simulink model "dyngeo"  (R2025b)
settings: Solver=VariableStepAuto  StartTime=0.0  StopTime=10.0  RelTol=1e-3
values from neighbouring files (symbols this model uses):
  g = 9.8    [initparams.m]
  I = diag([I_phi, I_theta, I_psi])    [initparams.m]
  m = 2.0    (= 2)    [initparams.m]
undefined symbols (not defined in the file or in its folder): Sim3dSensor
libraries: sim3dlib x2, uavsim3dlib x1, sim3dcameralib x1
settings Model: Creator=Sunetra  LastModifiedBy=Sunetra

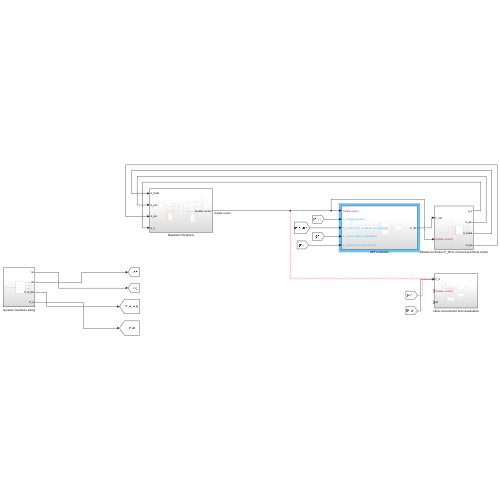
[thumbnail: Simulink's stored preview of the top-level diagram]
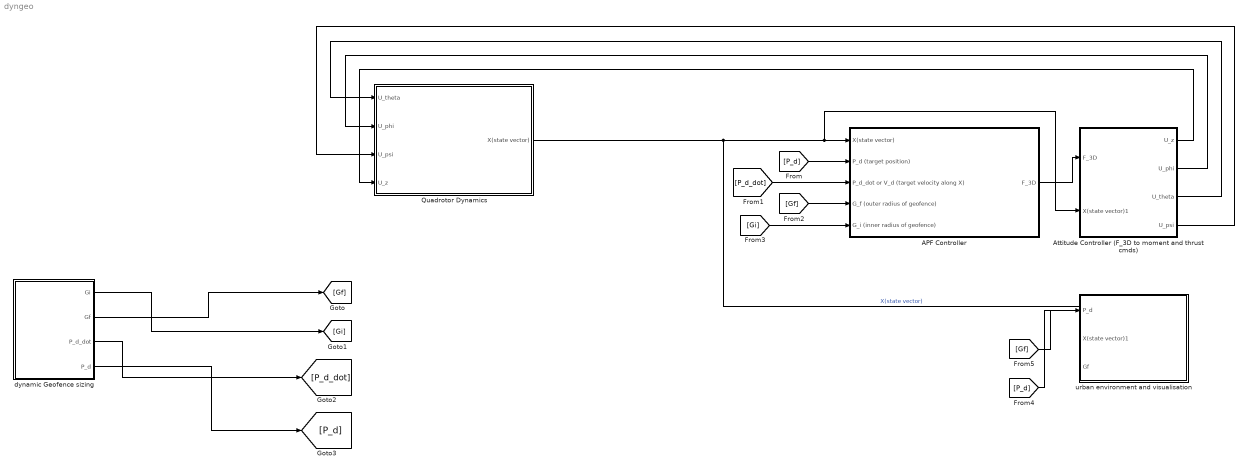
== system dyngeo ==
  APF Controller : Subsystem
  Attitude Controller (F_3D to moment and thrust cmds) : Subsystem
  Quadrotor Dynamics : Subsystem
  dynamic Geofence sizing : Subsystem
  urban environment and visualisation : Subsystem
  wires:
  Quadrotor Dynamics/1(X(state vector)) -> Attitude Controller (F_3D to moment and thrust cmds)/2(X(state vector)1), APF Controller/1(X(state vector))  "X(state vector)"
  APF Controller/1(F_3D) -> Attitude Controller (F_3D to moment and thrust cmds)/1(F_3D)
  Attitude Controller (F_3D to moment and thrust cmds)/1(U_z) -> Quadrotor Dynamics/4(U_z)
  Attitude Controller (F_3D to moment and thrust cmds)/2(U_phi) -> Quadrotor Dynamics/2(U_phi)
  Attitude Controller (F_3D to moment and thrust cmds)/3(U_theta) -> Quadrotor Dynamics/1(U_theta)
  Attitude Controller (F_3D to moment and thrust cmds)/4(U_psi) -> Quadrotor Dynamics/3(U_psi)
  dynamic Geofence sizing/2(Gf) -> [Gf]
  dynamic Geofence sizing/1(Gi) -> [Gi]
  dynamic Geofence sizing/3(P_d_dot) -> [P_d_dot]
  dynamic Geofence sizing/4(P_d) -> [P_d]
  [Gi] -> APF Controller/5(G_i (inner radius of geofence))
  [Gf] -> APF Controller/4(G_f (outer radius of geofence))
  [P_d_dot] -> APF Controller/3(P_d_dot or V_d (target velocity along X))
  [P_d] -> APF Controller/2(P_d (target position))
  [P_d] -> urban environment and visualisation/1(P_d)
  [Gf] -> ?

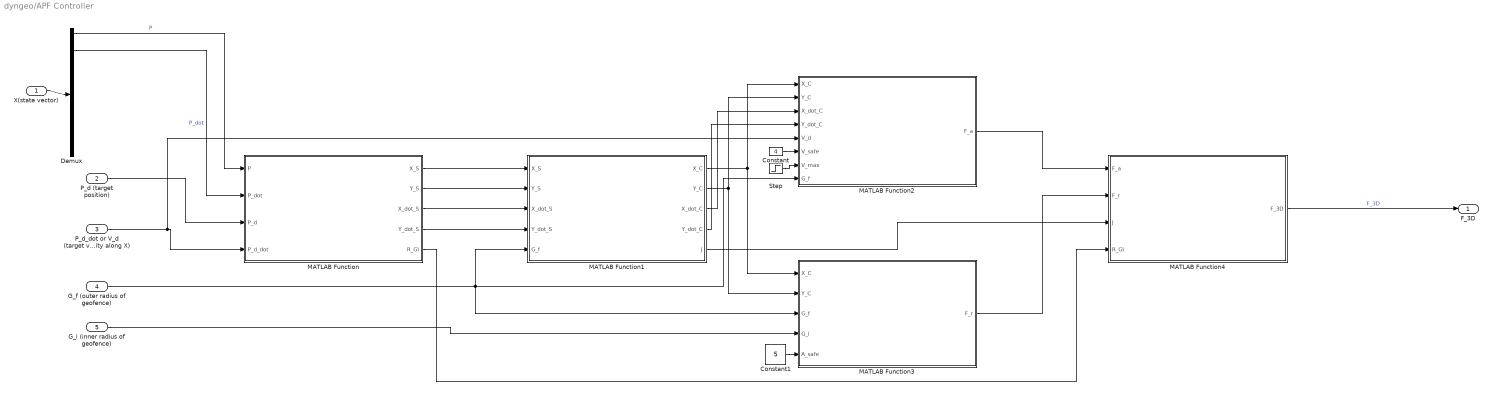
== system dyngeo/APF Controller ==
  X(state vector) : Inport
  P_d (target position) : Inport  Port=2
  P_d_dot or V_d (target velocity along X) : Inport  Port=3
  G_f (outer radius of geofence) : Inport  Port=4
  G_i (inner radius of geofence) : Inport  Port=5
  Constant : Constant  Value=4
  Constant1 : Constant  Value=5
  Demux : Demux  Outputs=[3, 3, 1, 1, 1, 1, 1, 1]
  MATLAB Function : MATLAB Function  TreatAsAtomicUnit=on
  MATLAB Function1 : MATLAB Function  TreatAsAtomicUnit=on
  MATLAB Function2 : MATLAB Function  TreatAsAtomicUnit=on
  MATLAB Function3 : MATLAB Function  TreatAsAtomicUnit=on
  MATLAB Function4 : MATLAB Function  TreatAsAtomicUnit=on
  Step : Step  Time=10  After=4  SampleTime=0
  F_3D : Outport
  wires:
  X(state vector)/1 -> Demux/1
  P_d (target position)/1 -> MATLAB Function/3(P_d)
  P_d_dot or V_d (target velocity along X)/1 -> MATLAB Function2/5(V_d), MATLAB Function/4(P_d_dot)
  Demux/1 -> MATLAB Function/1(P)  "P"
  Demux/2 -> MATLAB Function/2(P_dot)  "P_dot"
  MATLAB Function/1(X_S) -> MATLAB Function1/1(X_S)
  MATLAB Function/2(Y_S) -> MATLAB Function1/2(Y_S)
  MATLAB Function/3(X_dot_S) -> MATLAB Function1/3(X_dot_S)
  MATLAB Function/4(Y_dot_S) -> MATLAB Function1/4(Y_dot_S)
  G_f (outer radius of geofence)/1 -> MATLAB Function2/8(G_f), MATLAB Function3/3(G_f), MATLAB Function1/5(G_f)
  MATLAB Function1/1(X_C) -> MATLAB Function3/1(X_C), MATLAB Function2/1(X_C)
  MATLAB Function1/2(Y_C) -> MATLAB Function3/2(Y_C), MATLAB Function2/2(Y_C)
  MATLAB Function1/3(X_dot_C) -> MATLAB Function2/3(X_dot_C)
  MATLAB Function1/4(Y_dot_C) -> MATLAB Function2/4(Y_dot_C)
  G_i (inner radius of geofence)/1 -> MATLAB Function3/4(G_i)
  MATLAB Function2/1(F_a) -> MATLAB Function4/1(F_a)
  MATLAB Function3/1(F_r) -> MATLAB Function4/2(F_r)
  MATLAB Function1/5(J) -> MATLAB Function4/3(J)
  MATLAB Function/5(R_GI) -> MATLAB Function4/4(R_GI)
  MATLAB Function4/1(F_3D) -> F_3D/1  "F_3D"
  Constant/1 -> MATLAB Function2/6(V_safe)
  Step/1 -> MATLAB Function2/7(V_max)
  Constant1/1 -> MATLAB Function3/5(A_safe)

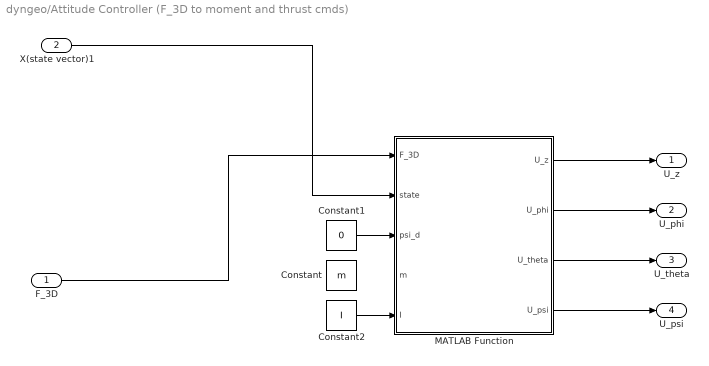
== system dyngeo/Attitude Controller (F_3D to moment and thrust cmds) ==
  F_3D : Inport
  X(state vector)1 : Inport  Port=2
  Constant : Constant  Value=m
  Constant1 : Constant  Value=0
  Constant2 : Constant  Value=I
  MATLAB Function : MATLAB Function  TreatAsAtomicUnit=on
  U_z : Outport
  U_phi : Outport  Port=2
  U_theta : Outport  Port=3
  U_psi : Outport  Port=4
  wires:
  F_3D/1 -> MATLAB Function/1(F_3D)
  X(state vector)1/1 -> MATLAB Function/2(state)
  Constant1/1 -> MATLAB Function/3(psi_d)
  Constant2/1 -> MATLAB Function/5(I)
  MATLAB Function/4(U_psi) -> U_psi/1
  MATLAB Function/3(U_theta) -> U_theta/1
  MATLAB Function/2(U_phi) -> U_phi/1
  MATLAB Function/1(U_z) -> U_z/1

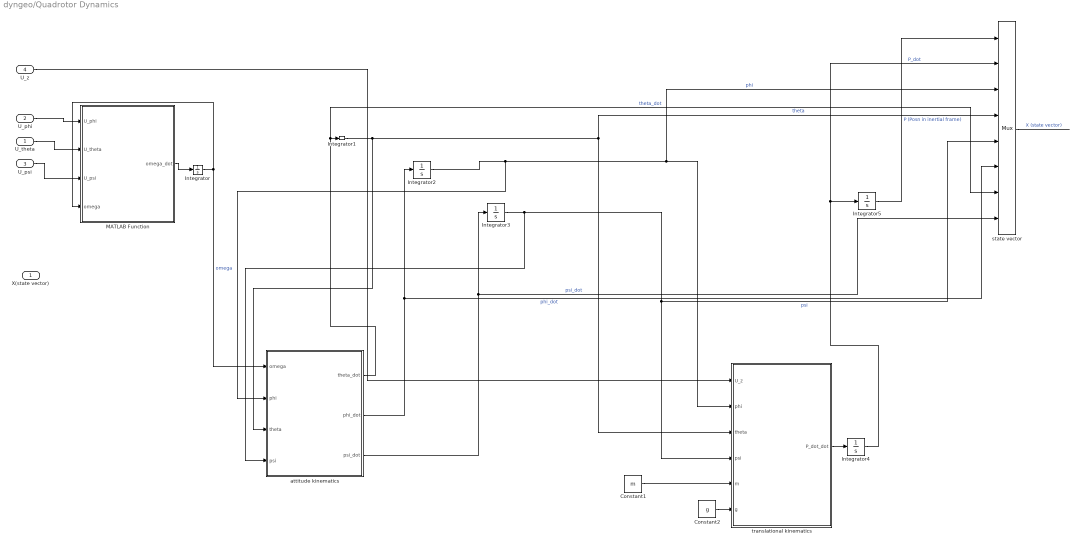
== system dyngeo/Quadrotor Dynamics ==
  U_theta : Inport
  U_phi : Inport  Port=2
  U_psi : Inport  Port=3
  U_z : Inport  Port=4
  Constant1 : Constant  Value=m
  Constant2 : Constant  Value=g
  Integrator : Integrator  InitialCondition=[0;0;0]
  Integrator{1..4} (4 alike) : Integrator
  Integrator5 : Integrator  InitialCondition=[0;0;0]
  MATLAB Function : MATLAB Function  TreatAsAtomicUnit=on
  attitude kinematics : MATLAB Function  TreatAsAtomicUnit=on
  "state vector " : Mux  Inputs=[3, 3, 1, 1, 1, 1, 1, 1]
  translational kinematics : MATLAB Function  TreatAsAtomicUnit=on
  X(state vector) : Outport
  wires:
  U_theta/1 -> MATLAB Function/2(U_theta)
  U_psi/1 -> MATLAB Function/3(U_psi)
  MATLAB Function/1(omega_dot) -> Integrator/1
  Integrator/1 -> MATLAB Function/4(omega), attitude kinematics/1(omega)  "omega"
  attitude kinematics/1(theta_dot) -> "state vector "/7, Integrator1/1  "theta_dot"
  attitude kinematics/2(phi_dot) -> Integrator2/1, "state vector "/6  "phi_dot"
  attitude kinematics/3(psi_dot) -> Integrator3/1, "state vector "/8  "psi_dot"
  Integrator2/1 -> attitude kinematics/2(phi), "state vector "/3, translational kinematics/2(phi)  "phi"
  Integrator3/1 -> attitude kinematics/4(psi), "state vector "/5, translational kinematics/4(psi)  "psi"
  Constant1/1 -> translational kinematics/5(m)
  Constant2/1 -> translational kinematics/6(g)
  translational kinematics/1(P_dot_dot) -> Integrator4/1
  Integrator4/1 -> "state vector "/2, Integrator5/1  "P_dot"
  Integrator5/1 -> "state vector "/1  "P (Posn in inertial frame)"
  Integrator1/1 -> attitude kinematics/3(theta), "state vector "/4, translational kinematics/3(theta)  "theta"
  U_phi/1 -> MATLAB Function/1(U_phi)
  U_z/1 -> translational kinematics/1(U_z)
  "state vector "/1 -> ?  "X (state vector)"

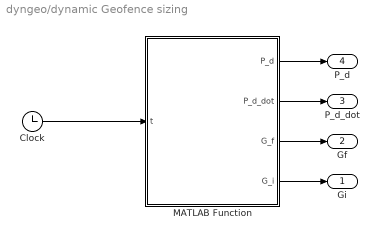
== system dyngeo/dynamic Geofence sizing ==
  Clock : Clock
  MATLAB Function : MATLAB Function  TreatAsAtomicUnit=on
  Gi : Outport
  Gf : Outport  Port=2
  P_d_dot : Outport  Port=3
  P_d : Outport  Port=4
  wires:
  Clock/1 -> MATLAB Function/1(t)
  MATLAB Function/1(P_d) -> P_d/1
  MATLAB Function/2(P_d_dot) -> P_d_dot/1
  MATLAB Function/3(G_f) -> Gf/1
  MATLAB Function/4(G_i) -> Gi/1

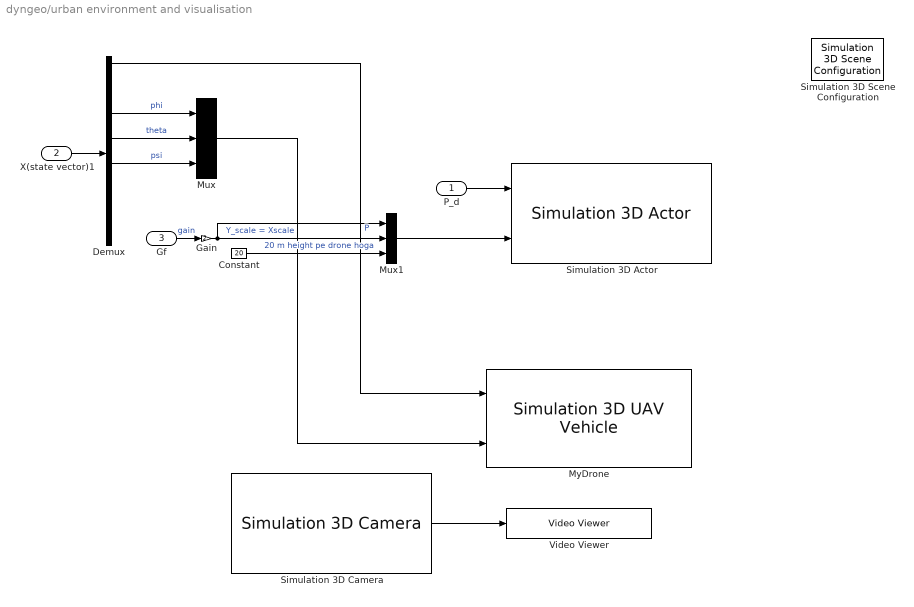
== system dyngeo/urban environment and visualisation ==
  P_d : Inport
  X(state vector)1 : Inport  Port=2
  Gf : Inport  Port=3
  Constant : Constant  Value=20
  Demux : Demux  Outputs=[3, 3, 1, 1, 1, 1, 1, 1]
  Gain : Gain  Gain=2
  Mux : Mux  Inputs=3
  Mux1 : Mux  Inputs=3
  MyDrone : uavsim3dlib/Simulation 3D UAV Vehicle  Priority=-1  Mesh=Quadrotor  MeshPath=/MathWorksUAVContent/UAVs/HexaRotorUAV/HexaRotor.HexaRotor  Color=Black  ActorName=MyDrone  UseGlobalFrame=off  InitialTranslation=[0 0 0]  InitialRotation=[0 0 0]  InitialTranslationGlobal=[0 0 0]  InitialGeoOrigin=[0 0 0]  InitialRotationGlobal=[0 0 0]  SampleTime=-1  ActorType=SimulinkVehicle  ID=C  aMode=4  ActorTag=MyDrone
  Simulation 3D Actor : sim3dlib/Simulation 3D Actor  Priority=1  ActorName=Sim3dActor1  ParentName=Scene Origin  Operation=Create at setup  InitScriptText=|  SampleTime=-1  Translation=[0 0 0]  Rotation=[0 0 0]  Scale=[1 1 1]  InputsText=Sim3dActor1.Translation Sim3dActor1.Scale  aMode=5  ActorTag=Sim3dActor1  ActorType=Sim3dActor  ID=1
      | % Reserved keywords:
      | % - Actor : handle to this actor object
      | % - World : handle to the world object
      | 
      | % Examples:
      | 
      | % Create a primitive geometry (optional)
      | % createShape(Actor, 'box', [1 1 1]);
      | 
      | % Initialize values (optional)
      | % Actor.Physics = true;
      | % Actor.Color = [1 0 0];
  Simulation 3D Camera : sim3dcameralib/Simulation 3D Camera  Priority=1  sensorTag=Sim3dSensor�  sensorId=1  sensorName=Sim3dSensor�  vehTagList={'MyDrone';'Scene Origin';'Sim3dActor1'}  vehTag=MyDrone  CoordinateSystem=ISO8855  mountLoc=Origin  offsetFlag=on  tmountOffset=[0, 0, 0]  extTmount=off  rmountOffset=[0, 0, 0]  extRmount=off  FocalLength=[1109, 1109]  OpticalCenter=[640, 360]  ImageSize=[720, 1280]  RadialDistortion=[0, 0]  TangentialDistortion=[0, 0]  SensorSkew=0  VisualizeFieldOfView=off  FieldOfViewRange=61  DepthOutportEnabled=off  SemanticOutportEnabled=off  TransformOutportEnabled=off  SampleTime=-1  mountPoint=[0 0 0]  mountOrientation=[0 0 0]  aMode=6  ID=1
      settings: LibrarySourceBlock=robotsim3dlib/Simulation 3D Camera
  Simulation 3D Scene Configuration : sim3dlib/Simulation 3D Scene Configuration  Priority=0  ProjectFormat=Default Scenes  SceneDesc=US city block  ProjectName=D:\MATLAb\toolbox\shared\sim3d_projects\automotive_project_windows\UE\WindowsNoEditor\VehicleSimulation.exe  ScenePath=/Game/Maps/HwStrght  EnableOpenDRIVE=off  vehTagList={'Custom';'MyDrone';'Scene Origin';'Sim3dActor1'}  vehTag=MyDrone  AttachedCameraRelativeTranslation=[0 0 0]  FreeCameraDefaultInitialTranslation=[-6, 0, 2]  AttachedCameraRelativeRotation=[0 0 0]  FreeCameraDefaultInitialRotation=[0, -15, 0]  ViewpointName=Custom  FreeCameraInitialTranslation=[-6, 0, 2]  ViewpointTranslation=[0 0 0]  FreeCameraInitialRotation=[0, -15, 0]  ViewpointRotation=[0 0 0]  OpVisEn=off  Ts=.02  EnableWindow=on  EnableRemoteAccess=off  EnableWeather=off  SunAzimuth=90  SunAltitude=40.0  EnableGeospatialSun=off  Latitude=0  Longitude=0  Date=2023-01-01  Time=10:30:00  GeoTimeZone=-5.0  SunDaylightSaving=off  wind=1  clouds=10  EnableVolumetricClouds=off  CloudCoverage=0  CloudAltitude=6  fog=0  rain=0  RaindropsEffect=off  SnowDensity=0  EnableGeospatial=off  TilesetSource=Earth terrain  UseTrueOrigin=off  OriginHeight=200  OriginLatitude=40.744652  OriginLongitude=-73.988864  MapStyle=Aerial  AdditionalAssetIDs=[]  UseAdvancedSunSky=off  SolarTime=11  TimeZone=-5  Day=21  Month=9  Year=2022  UseDaylightSavingTime=on  DSTStartDay=10  DSTStartMonth=3  DSTEndDay=3  DSTEndMonth=11  DSTSwitchHour=2  sensorTag=MainCamera1  sensorId=1  sensorName=MainCamera1  mountLoc=Origin  offsetFlag=off  tmountOffset=[0, 0, 0]  rmountOffset=[0, 0, 0]  HorizontalResolution=1280  VerticalResolution=720  HorizontalFOV=60  mountPoint=[0 0 0]  mountOrientation=[0 0 0]  aMode=0  ID=1  GeoTrigger=Inactive  ViewNameList={'Custom'}  ViewTranslationList={'[-6 0 2]'}  ViewRotationList={'[0 -15 0]'}
      settings: LibrarySourceBlock=aerolibsim3d/Simulation 3D Scene Configuration
  Video Viewer : VideoViewer  FigPos=[2041 741 418 304]
  wires:
  Demux/1 -> MyDrone/1  "P"
  X(state vector)1/1 -> Demux/1
  Demux/4 -> Mux/2  "theta"
  Demux/5 -> Mux/3  "psi"
  Demux/3 -> Mux/1  "phi"
  Mux/1 -> MyDrone/2
  P_d/1 -> Simulation 3D Actor/1
  Mux1/1 -> Simulation 3D Actor/2
  Gain/1 -> Mux1/2, Mux1/1  "Y_scale = Xscale"
  Constant/1 -> Mux1/3  "20 m height pe drone hoga"
  Gf/1 -> Gain/1  "gain"
  Simulation 3D Camera/1 -> Video Viewer/1

== matlab function dyngeo/APF Controller/MATLAB Function4 ==
  data: F_a input; F_3D output; F_r input; J input; R_GI input
function F_3D = inverse_mapping_2D23D(F_a, F_r, J, R_GI)
    % Inputs:
    % F_a, F_r : 2D force vectors from the Attractive and Repulsive fields
    % J        : 2x2 Jacobian matrix (from the Forward Mapping block)
    % R_GI     : 3x3 Rotation matrix (from the 3D to 2D Transform block)
    
    % Outputs:
    % F_3D     : 3x1 Commanded acceleration vector [U_x; U_y; U_z] in the inertial frame

    % 1. Calculate the net planar field
    F_planar = F_a + F_r;
    
    % 2. Invert the 2x2 Jacobian
    % We use a determinant check to prevent singular matrix errors 
    % at the extreme mathematical boundaries of the diffeomorphic map.
    if abs(det(J)) > 1e-6
        J_inv = inv(J);
    else
        J_inv = pinv(J); % Moore-Penrose pseudo-inverse as a numerical safety net
    end
    
    % 3. Construct the 3D Inverse Jacobian mapping (Equation 6)
    % The Z-axis remains unchanged (1) because the diffeomorphic map only squishes the X-Y plane
    J_inv_3D = [J_inv(1,1), J_inv(1,2), 0;
                J_inv(2,1), J_inv(2,2), 0;
                0,          0,          1];
                
    % 4. Pad the 2D planar force to 3D
    % The force is purely lateral in the cross-section, so Z is 0
    F_padded = [F_planar(1); F_planar(2); 0];
    
    % 5. Map the force back to the square cross-section
    F_square = J_inv_3D * F_padded;
    
    % 6. Rotate the force back to the 3D Inertial Frame (Equation 6)
    % Since R_GI is an orthogonal rotation matrix, its pseudo-inverse (dagger) 
    % is simply its transpose (R_GI').
    F_3D = R_GI' * F_square;
    
end

== matlab function dyngeo/Attitude Controller (F_3D to moment and thrust cmds)/MATLAB Function ==
  data: F_3D input; U_z output; state input; psi_d input; m input; I input; U_phi output; U_theta output; U_psi output
function [U_z, U_phi, U_theta, U_psi] = attitude_controller(F_3D, state, psi_d, m, I)
    % Inputs:
    % F_3D   : 3x1 Commanded acceleration vector from APF [U_x; U_y; U_z_accel]
    % state  : 12x1 State vector from Quadrotor [P; P_dot; phi; theta; psi; phi_dot; theta_dot; psi_dot]
    % psi_d  : Desired heading angle (rad)
    % m      : Mass (kg)
    % I      : 3x3 Inertia matrix
    
    % Outputs:
    % U_z    : Total thrust force command (N)
    % U_phi  : Roll moment command (Nm)
    % U_theta: Pitch moment command (Nm)
    % U_psi  : Yaw moment command (Nm)

    g = 9.8;

    % --- 1. Extract Current States ---
    % Assuming your state vector is packed as [P(1:3); P_dot(1:3); Euler(1:3); Euler_rates(1:3)]
    phi       = state(7);
    theta     = state(8);
    psi       = state(9);
    phi_dot   = state(10);
    theta_dot = state(11);
    psi_dot   = state(12);

    % --- 2. Force Allocation & Desired Angles (Eq A1 & A2) ---
    U_x = F_3D(1);
    U_y = F_3D(2);
    
    % Total thrust must counteract gravity and provide the Z acceleration
    U_z_accel = F_3D(3) + g; 
    
    % Convert commanded acceleration to total thrust force
    % We use max(0, ...) to ensure the drone cannot command "negative" pulling thrust
    U_z = m * max(0, U_z_accel);

    % Calculate desired roll and pitch angles to achieve U_x and U_y accelerations
    phi_d   = (U_x * sin(psi_d) - U_y * cos(psi_d)) / g;
    theta_d = (U_x * cos(psi_d) + U_y * sin(psi_d)) / g;

    % --- 3. PD Controller Gains ---
    % Sourced directly from the paper's tuning parameters
    
    % Roll and Pitch dynamics: damping ratio = 0.85, natural frequency = 14 rad/s
    zeta_rp = 0.85;
    wn_rp   = 14;
    
    % Yaw dynamics: damping ratio = 0.95, natural frequency = 18 rad/s
    zeta_y  = 0.95;
    wn_y    = 18;

    % --- 4. Calculate Control Moments (Eq A3) ---
    % U = Kp*(angle_d - angle) - Kv*(angle_dot)
    % where Kp = I * wn^2 and Kv = I * 2 * zeta * wn
    
    I_phi   = I(1,1);
    I_theta = I(2,2);
    I_psi   = I(3,3);

    % Roll Moment
    Kp_phi = I_phi * wn_rp^2;
    Kv_phi = I_phi * 2 * zeta_rp * wn_rp;
    U_phi  = Kp_phi * (phi_d - phi) - Kv_phi * phi_dot;

    % Pitch Moment
    Kp_theta = I_theta * wn_rp^2;
    Kv_theta = I_theta * 2 * zeta_rp * wn_rp;
    U_theta  = Kp_theta * (theta_d - theta) - Kv_theta * theta_dot;

    % Yaw Moment
    Kp_psi = I_psi * wn_y^2;
    Kv_psi = I_psi * 2 * zeta_y * wn_y;
    U_psi  = Kp_psi * (psi_d - psi) - Kv_psi * psi_dot;

end

== matlab function dyngeo/dynamic Geofence sizing/MATLAB Function ==
  data: t input; P_d output; P_d_dot output; G_f output; G_i output
function [P_d, P_d_dot, G_f, G_i] = mission_planner(t)

%To keep the model clean, this block will simultaneously calculate 
% the geofence sizes and generate the moving target position 
% (P_d) for the drone to chase.

%For this specific setup, the guidance logic simplifies significantly 
% because the path is a straight line. Since the curvature is zero, 
% you don't need the dynamic "breathing" behavior of the safety envelopes 
% that you would see during complex turns. Instead, the inner boundary 
% stays fixed relative to the outer boundary.

%For this initial setup, we will use the parameters 
% from Case 4 in the paper: a worst-case, head-on wind disturbance 
% ($\alpha_{max} = 180^\circ$) on a straight-line path. 
% Because a straight-line path has zero curvature, 
% the paper states (Equation 85) that the inner radius $G_i$ should simply 
% sit at $0.99 G_f$ to act as a static safety bumper, 
% rather than constantly expanding and shrinking.

% Inputs:
    % t       : Current simulation time (seconds)
    
    % Outputs:
    % P_d     : 3x1 Desired position vector
    % P_d_dot : 3x1 Desired velocity vector
    % G_f     : Outer geofence radius (m)
    % G_i     : Inner geofence radius (m)

    % --- 1. Mission & Wind Parameters (Case 4) ---
    V_d = 2.0;          % Desired flight speed (m/s)
    V_safe = 4.0;       % Drone's safe speed limit (m/s)
    V_max = 4.0;        % Max speed induced by worst-case wind (m/s)
    alpha_max = pi;     % Wind direction (180 deg = head-on wind)

    % APF Tuning Gains (sourced from paper)
    K_p = 0.0905;
    K_v = 0.4254;
    K_m = 1.0;          % Lyapunov stability gain

    % --- 2. Calculate Wind Perturbation (Equation 22) ---
    delta_V = sqrt((V_max*cos(alpha_max) - V_d)^2 + (V_max*sin(alpha_max))^2);

    % --- 3. Calculate Dynamic Shift Parameters ---
    K_a = V_max / V_d;
    mu = K_v / (K_p * K_a);

    % --- 4. Theorem 2: Geofence Sizing (Equations 20 & 21) ---
    % This calculates the minimum safe G_radius based on the Lyapunov bounds
    term1 = (K_m * delta_V^2 / K_v) / (1 + K_m / mu);
    term2 = mu * (V_safe - V_d);

    if sqrt(term1) < term2
        G_f = sqrt(term1);
    else
        % Eq 21: Expanding the quadratic root
        G_f = 0.5 * (-K_m*(V_safe - V_d) + sqrt((K_m*(V_safe - V_d))^2 + 4*(K_m*delta_V^2/K_v)));
    end

    % --- 5. Inner Radius (Equation 85 Logic) ---
    % For a straight path (curvature c(t) = 0), G_i is fixed near the outer wall
    G_i = 0.99 * G_f;

    % --- 6. Path Generation (Straight Line along X-axis) ---
    P_d = [V_d * t; 0; 0];
    P_d_dot = [V_d; 0; 0];
    
end

== matlab function dyngeo/Quadrotor Dynamics/attitude kinematics ==
  data: omega input; phi input; theta input; psi input; theta_dot output; phi_dot output; psi_dot output
function [theta_dot, phi_dot,psi_dot] = attitude_kinematics(omega,phi,theta, psi)

% Inputs:
    % omega : Angular velocity [p; q; r] (rad/s) in body frame
    % phi   : Roll angle (rad)
    % theta : Pitch angle (rad)
    % psi   : Yaw angle (rad)
    
    % Outputs:
    % phi_dot   : Roll rate (rad/s)
    % theta_dot : Pitch rate (rad/s)
    % psi_dot   : Yaw rate (rad/s)

    % Define the transformation matrix from Equation A5
    W = [cos(theta), 0, -cos(phi)*sin(theta);
         0,          1,  sin(phi);
         sin(theta), 0,  cos(phi)*cos(theta)];
         
    % Calculate Euler rates: [phi_dot; theta_dot; psi_dot] = W^-1 * omega
    % Using the backslash operator (\) for efficient matrix inversion
    euler_rates = W \ omega;
    
    % Extract individual rates for the output ports
    phi_dot   = euler_rates(1);
    theta_dot = euler_rates(2);
    psi_dot   = euler_rates(3);
end

== matlab function dyngeo/Quadrotor Dynamics/MATLAB Function ==
  data: U_phi input; omega_dot output; U_theta input; U_psi input; omega input
function omega_dot = rotational_dynamics(U_phi, U_theta, U_psi, omega)

    % Pull I directly from workspace as a parameter
    I = diag([0.0196, 0.0196, 0.0264]); % hardcode or match your workspace values

    omega = omega(:);  % ensure 3x1

    M = [U_phi; U_theta; U_psi];

    omega_dot = I \ (M - cross(omega, I * omega));
end

== matlab function dyngeo/Quadrotor Dynamics/translational kinematics ==
  data: U_z input; P_dot_dot output; phi input; theta input; psi input; m input; g input
function P_dot_dot   = translational_physics(U_z,phi, theta, psi, m, g)

% Inputs:
    % U_z   : Total thrust command (N)
    % phi   : Roll angle (rad)
    % theta : Pitch angle (rad)
    % psi   : Yaw angle (rad)
    % m     : Mass (kg) sourced from workspace
    % g     : Gravity (m/s^2) sourced from workspace
    
    % Outputs:
    % P_dot_dot : Linear acceleration [x_ddot; y_ddot; z_ddot] in inertial frame

    % 1. Construct the Z-Y-X Rotation Matrix (R^BN) from Equation A6
    % Row 1
    R11 = cos(theta)*cos(psi);
    R12 = cos(psi)*sin(theta)*sin(phi) - sin(psi)*cos(phi);
    R13 = cos(psi)*sin(theta)*cos(phi) + sin(psi)*sin(phi);
    
    % Row 2
    R21 = sin(psi)*cos(theta);
    R22 = sin(psi)*sin(theta)*sin(phi) + cos(psi)*cos(phi);
    R23 = sin(psi)*sin(theta)*cos(phi) - cos(psi)*sin(phi);
    
    % Row 3
    R31 = -sin(theta);
    R32 = cos(theta)*sin(phi);
    R33 = cos(theta)*cos(phi);
    
    R_BN = [R11, R12, R13; 
            R21, R22, R23; 
            R31, R32, R33];
            
    % 2. Implement Position Dynamics from Equation A7
    gravity_vector = [0; 0; -g];
    
    % The thrust acts purely along the body Z-axis.
    % Dividing U_z by m converts force (Newtons) to acceleration (m/s^2)
    thrust_vector = [0; 0; U_z / m]; 
    
    % Calculate final linear acceleration
    P_dot_dot = gravity_vector + (R_BN * thrust_vector);
end

== matlab function dyngeo/APF Controller/MATLAB Function ==
  data: P input; X_S output; P_dot input; P_d input; P_d_dot input; Y_S output; X_dot_S output; Y_dot_S output; R_GI output
function [X_S, Y_S, X_dot_S, Y_dot_S, R_GI] = frame_transform_3D_to_2D(P, P_dot, P_d, P_d_dot)
    % Inputs:
    % P, P_dot       : Current UAS 3D position and velocity (3x1 vectors)
    % P_d, P_d_dot   : Desired 3D position and velocity on the path (3x1 vectors)
    
    % Outputs:
    % X_S, Y_S       : 2D Relative position in the square cross-section
    % X_dot_S, Y_dot_S : 2D Relative velocity in the square cross-section
    % R_GI           : 3x3 Rotation matrix (Save this to map forces back to 3D later)

    % Ensure inputs are column vectors for matrix operations
    P = P(:); P_dot = P_dot(:); P_d = P_d(:); P_d_dot = P_d_dot(:);
    
    % 1. Calculate relative 3D position and velocity
    del_P = P - P_d;
    del_P_dot = P_dot - P_d_dot;
    
    % 2. Path tangent vector (X_hat) [cite: 299]
    v_d_norm = norm(P_d_dot);
    if v_d_norm > 1e-6
        X_hat = P_d_dot / v_d_norm;
    else
        X_hat = [1; 0; 0]; % Fallback if desired velocity drops to exact 0
    end
    
    % 3. Intermediate frame vectors (Y_i_hat, Z_i_hat) [cite: 300, 301]
    Y_i_hat = [0; 1; 0];
    cross_X_Yi = cross(X_hat, Y_i_hat);
    if norm(cross_X_Yi) > 1e-6
        Z_i_hat = cross_X_Yi / norm(cross_X_Yi);
    else
        Z_i_hat = [0; 0; 1]; % Fallback if path is perfectly vertical
        Y_i_hat = cross(Z_i_hat, X_hat);
    end
    
    % 4. Geofence frame vectors (Z_g_hat, Y_g_hat) [cite: 301, 302]
    cross_X_delP = cross(X_hat, del_P);
    
    % Singularity handling: If drone is exactly on the centerline, cross product is 0
    if norm(cross_X_delP) > 1e-6
        Z_g_hat = cross_X_delP / norm(cross_X_delP);
        Y_g_hat = cross(Z_g_hat, X_hat) / norm(cross(Z_g_hat, X_hat));
    else
        % Align Geofence frame with Intermediate frame to avoid divide-by-zero
        Z_g_hat = Z_i_hat;
        Y_g_hat = Y_i_hat;
    end
    
    % 5. Construct the Rotation Matrix [R_GI] (Equation 4) [cite: 306]
    e1 = [1; 0; 0];
    M_i = [e1, Y_i_hat, Z_i_hat];
    M_g = [X_hat, Y_g_hat, Z_g_hat];
    
    % R_GI = M_i * M_g^T
    R_GI = M_i * M_g'; 
    
    % 6. Apply rotation to get states in the square cross-section [cite: 306]
    P_S_3D = R_GI * del_P;
    P_S_dot_3D = R_GI * del_P_dot;
    
    % 7. Extract the 2D planar components (We only care about the X and Y plane here)
    X_S = P_S_3D(1);
    Y_S = P_S_3D(2);
    X_dot_S = P_S_dot_3D(1);
    Y_dot_S = P_S_dot_3D(2);
end

== matlab function dyngeo/APF Controller/MATLAB Function1 ==
  data: X_C output; X_S input; Y_S input; X_dot_S input; Y_dot_S input; Y_C output; X_dot_C output; Y_dot_C output; J output; G_f input
function [X_C, Y_C, X_dot_C, Y_dot_C, J] = square2circle(X_S, Y_S, X_dot_S, Y_dot_S, G_f)
    % Inputs:
    % X_S, Y_S         : 2D position in the square cross-section
    % X_dot_S, Y_dot_S : 2D velocity in the square cross-section
    % G_f              : Outer geofence radius (G_radius)
    
    % Outputs:
    % X_C, Y_C         : 2D position in the circular manifold
    % X_dot_C, Y_dot_C : 2D velocity in the circular manifold
    % J                : 2x2 Jacobian matrix (passed forward for inverse mapping)

    % 1. Implement Equation 2 (Elliptical Grid Mapping)
    % We use max(0, ...) to prevent imaginary numbers if floating-point 
    % inaccuracies push the drone slightly past the absolute corner.
    term_Y = max(0, 1 - 0.5 * (Y_S / G_f)^2);
    term_X = max(0, 1 - 0.5 * (X_S / G_f)^2);
    
    X_C = X_S * sqrt(term_Y);
    Y_C = Y_S * sqrt(term_X);
    
    % 2. Calculate the Jacobian Matrix elements for velocity mapping
    % J11 = d(X_C)/d(X_S)
    J11 = sqrt(term_Y);
    
    % J12 = d(X_C)/d(Y_S)
    if term_Y > 1e-6
        J12 = - (X_S * Y_S) / (2 * G_f^2 * sqrt(term_Y));
    else
        J12 = 0; % Prevent divide-by-zero at extreme boundaries
    end
    
    % J21 = d(Y_C)/d(X_S)
    if term_X > 1e-6
        J21 = - (X_S * Y_S) / (2 * G_f^2 * sqrt(term_X));
    else
        J21 = 0;
    end
    
    % J22 = d(Y_C)/d(Y_S)
    J22 = sqrt(term_X);
    
    % Construct the 2x2 Jacobian
    J = [J11, J12; 
         J21, J22];
         
    % 3. Map the velocities into the circular manifold using the Jacobian
    V_C = J * [X_dot_S; Y_dot_S];
    
    X_dot_C = V_C(1);
    Y_dot_C = V_C(2);
end

== matlab function dyngeo/APF Controller/MATLAB Function2 ==
  data: X_C input; F_a output; Y_C input; X_dot_C input; Y_dot_C input; V_d input; V_safe input; V_max input; G_f input
function F_a = attractive_field(X_C, Y_C, X_dot_C, Y_dot_C, V_d, V_safe, V_max, G_f)
    % Outputs:
    % F_a : 2D Attractive force vector in the circular manifold
    
    % Internal Proportional and Derivative Gains 
    % (You can tune these later or expose them as block inputs)
    K_p = 0.0905; 
    K_v = 0.4254; 

    % Drone state relative to the desired position (which sits at [0;0] in this frame)
    Q = [X_C; Y_C];
    Q_dot = [X_dot_C; Y_dot_C];
    norm_Q = norm(Q);

    % If the drone is outside the outer geofence, F_a is mathematically 0 
    % (The repulsive field handles the extreme edge)
    if norm_Q > G_f
        F_a = [0; 0];
        return;
    end

    % 1. Calculate dynamic shift parameters
    K_a = V_max / V_d;
    mu = K_v / (K_p * K_a);

    % Path tangent vector in this rotated 2D frame is strictly along the X-axis
    X_hat = [1; 0];

    % 2. Calculate the zero-potential point (Q_d)
    % Initial assumption for shift X_E (Equation 15)
    X_E = mu * V_d;
    Q_d = X_E * X_hat;
    dist_Q_Qd = norm(Q - Q_d);

    % Check if the drone crossed the velocity boundary
    if dist_Q_Qd > mu * V_safe
        % Recalculate X_E dynamically to prevent exceeding safe speeds
        X_E = V_d * dist_Q_Qd / V_safe;
        Q_d = X_E * X_hat;
    end

    % 3. Calculate Reference Velocity (Equation 9)
    Q_d_dot = (K_p / K_v) * (Q_d - Q);
    norm_Q_d_dot = norm(Q_d_dot);

    if norm_Q_d_dot > 1e-6
        gamma = min(K_a, V_safe / norm_Q_d_dot);
    else
        gamma = K_a;
    end

    % 4. Compute Final Attractive Force (Equation 10)
    F_a = -K_v * (Q_dot - gamma * Q_d_dot);
end

== matlab function dyngeo/APF Controller/MATLAB Function3 ==
  data: X_C input; F_r output; Y_C input; G_f input; G_i input; A_safe input
function F_r = repulsive_field(X_C, Y_C, G_f, G_i, A_safe)
    % Outputs:
    % F_r : 2D Repulsive force vector in the circular manifold
    
    % Eta defines the fraction of A_safe reserved for the attractive field.
    % We assume 50% is reserved for path curvature here (eta = 0.5).
    eta = 0.5; 

    % Position vector
    Q = [X_C; Y_C];
    norm_Q = norm(Q);

    % Calculate signed distances (Equation 48 & 49)
    rho_i = G_i - norm_Q;
    rho = G_f - norm_Q;

    % Repulsive logic (Equation 52): 
    % Triggers ONLY if drone is in the annular region between G_i and G_f
    if (rho_i <= 0) && (rho >= 0) && (norm_Q > 1e-6) && (G_f > G_i)
        
        % The force directs inward, opposite to the drone's radial position
        direction = -Q / norm_Q;

        % Magnitude scales quadratically as the drone approaches G_f
        magnitude = (1 - eta) * A_safe * (-rho_i / G_f) * (-rho_i / (G_f - G_i));

        F_r = magnitude * direction;
    else
        F_r = [0; 0];
    end
end
